simulink model "COLQR_RLGA"  (R2024b)
settings: Solver=VariableStepAuto  StartTime=0.0  StopTime=10.0  RelTol=1e-3
values from neighbouring files (symbols this model uses):
  A = [A_top; A_bottom]    [Dynamic_model.m]    (also in WhaleOptimizationAlgorithm.m = evalin('base', 'A'))
  Bce = [Bc, E]    [Dynamic_model.m]
  C = [C_top; C_bottom]    [Dynamic_model.m]
  Dcf = [Dc, F]    [Dynamic_model.m]
  F_MR_MAX = 5.0 * 10^4    (= 50000)    [COLQR.m]    (also in RLGA_LQR_Optimizer.m = 20000; RLGA_RL_toolbox.m = 20000; WOA_Optimizer.m = 20000; WhaleOptimizationAlgorithm.m = evalin('base', 'F_MR_MAX'))
  F_MR_MIN = -F_MR_MAX    (= -50000)    [COLQR.m]    (also in COLQR_CostFunction.m = 0; RLGA_LQR_Optimizer.m = -20000; RLGA_RL_toolbox.m = -20000; WOA_Optimizer.m = 0)
  K_RLGA = lqr(A, Bc, Q_RLGA, R_RLGA)    [RLGA_LQR_Optimizer.m]    (also in RLGA_RL_toolbox.m)
settings Model: Creator=Arghya  LastModifiedBy=Arghya

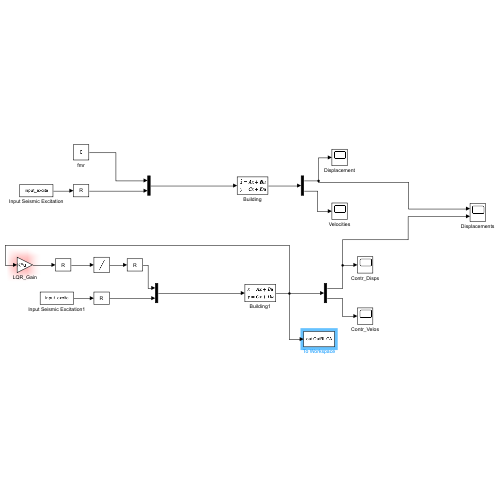
[thumbnail: Simulink's stored preview of the top-level diagram]
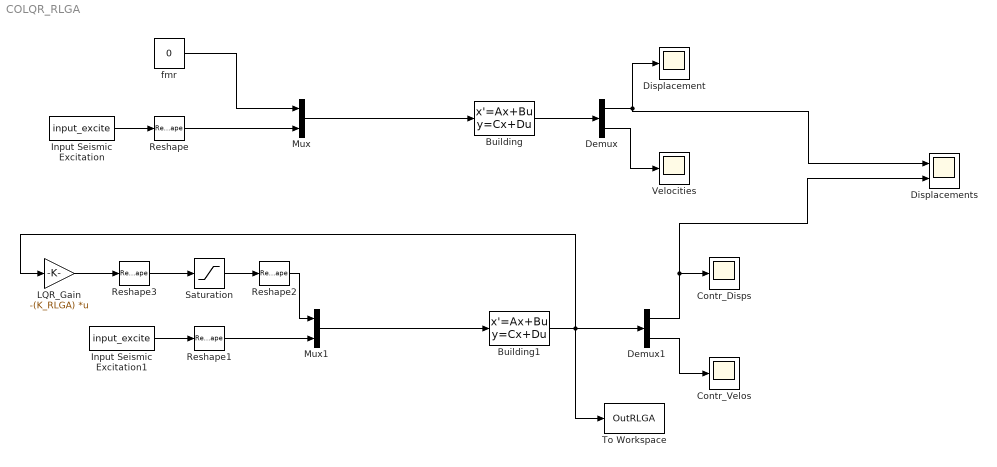
== system COLQR_RLGA ==
  Building : StateSpace  A=A  B=Bce  C=C  D=Dcf  InitialCondition=0  ContinuousStateAttributes="\"Building\""
  Building1 : StateSpace  A=A  B=Bce  C=eye(20)  D=zeros(20,2)  InitialCondition=0  ContinuousStateAttributes="\"Building\""
  Contr_Disps : Scope
  Contr_Velos : Scope
  Demux : Demux  Outputs=2
  Demux1 : Demux  Outputs=2
  Displacement : Scope
  Displacements : Scope  NumInputPorts=2
  Input Seismic Excitation : FromWorkspace  VariableName=input_excite  OutputAfterFinalValue=Setting to zero
  Input Seismic Excitation1 : FromWorkspace  VariableName=input_excite  OutputAfterFinalValue=Setting to zero
  LQR_Gain : Gain  Gain=-(K_RLGA)  Multiplication=Matrix(K*u)
  Mux : Mux  Inputs=2
  Mux1 : Mux  Inputs=2
  Reshape{,1..3} (4 alike) : Reshape  OutputDimensionality=Customize
  Saturation : Saturate  UpperLimit=F_MR_MAX  LowerLimit=F_MR_MIN
  To Workspace : ToWorkspace  VariableName=OutRLGA  SaveFormat=Timeseries  SampleTime=-1
  Velocities : Scope
  fmr : Constant  Value=0  SampleTime=0.002
  wires:
  Building/1 -> Demux/1
  fmr/1 -> Mux/1
  Demux/2 -> Velocities/1
  Input Seismic Excitation/1 -> Reshape/1
  Reshape/1 -> Mux/2
  Mux/1 -> Building/1
  Input Seismic Excitation1/1 -> Reshape1/1
  Reshape1/1 -> Mux1/2
  Mux1/1 -> Building1/1
  Building1/1 -> Demux1/1, LQR_Gain/1, To Workspace/1
  Saturation/1 -> Reshape2/1
  Reshape2/1 -> Mux1/1
  LQR_Gain/1 -> Reshape3/1
  Reshape3/1 -> Saturation/1
  Demux1/2 -> Contr_Velos/1
  Demux/1 -> Displacements/1, Displacement/1
  Demux1/1 -> Displacements/2, Contr_Disps/1
